simulink model "Kinematic_control"  (R2022b)
settings: Solver=FixedStepAuto  StartTime=0.0  StopTime=T_final  FixedStep=Ts  RelTol=1e-3
values from neighbouring files (symbols this model uses):
  BDD_thresh = 1    [Run_model.m]
  d = 0.1    [Run_model.m]
  I_single = sort(randperm(n_meas,n_attack)).'    [Run_model.m]
  kx = 15    [Run_model.m]
  ky = 15    [Run_model.m]
  max_iter = 2000    [Run_model.m]
  n_meas = 6    [Run_model.m]
  P_inp = 1e-10    [Run_model.m]
  R_meas = 1e-4    (= 0.0001)    [Run_model.m]
  Ts = 0.01    [Run_model.m]    (also in imu.m)
  u0 = zeros(n_int,1)    [Run_model.m]
  y0 = zeros(n_meas,1)    [Run_model.m]
  z_hat0 = z_initial    [Run_model.m]
  z_initial = [theta0;x0;y0]    [Run_model.m]
libraries: simulink x2, sharedTrackingLibrary x1
settings Model: Creator=Abelb  LastModifiedBy=Abelb

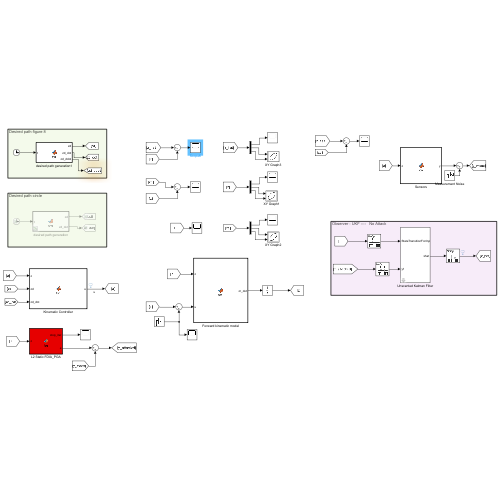
[thumbnail: Simulink's stored preview of the top-level diagram]
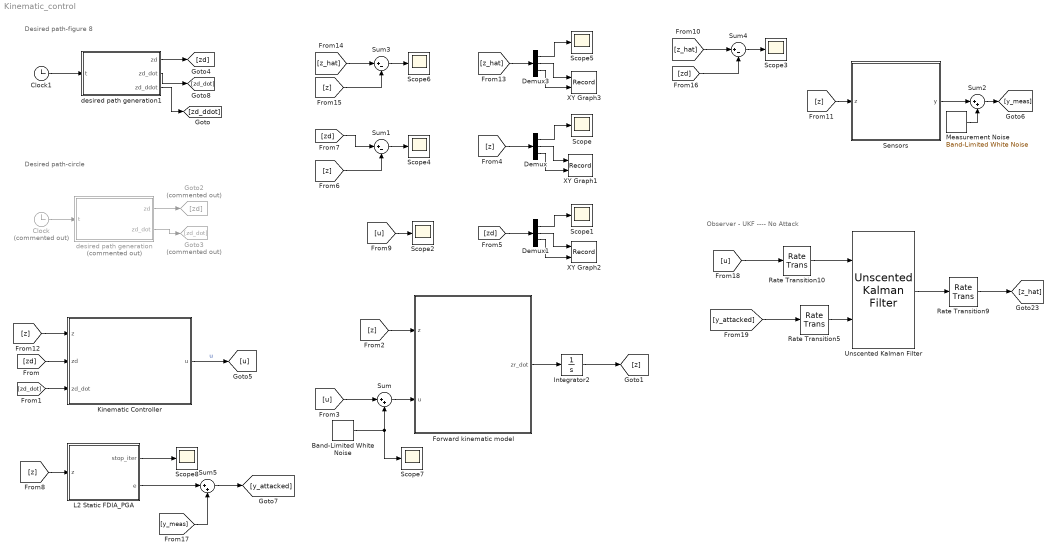
== system Kinematic_control ==
  note: Desired path-circle
  note: Desired path-figure 8
  note: Observer - UKF ---- No Attack
  Band-Limited White Noise : simulink/Sources/Band-Limited White Noise  Cov=P_inp*Ts  Ts=Ts  seed=[23341]
  Clock : Clock  Commented=on
  Clock1 : Clock
  Demux : Demux  Outputs=3
  Demux1 : Demux  Outputs=3
  Demux3 : Demux  Outputs=3
  Forward kinematic model : MATLAB Function  TreatAsAtomicUnit=on
  Goto2 : Goto  Commented=on  GotoTag=zd
  Goto3 : Goto  Commented=on  GotoTag=zd_dot
  Integrator2 : Integrator  InitialCondition=z_initial
  Kinematic Controller : MATLAB Function  TreatAsAtomicUnit=on
  L2 Static FDIA_PGA : MATLAB Function  TreatAsAtomicUnit=on
  Measurement Noise : simulink/Sources/Band-Limited White Noise  Cov=R_meas*Ts  Ts=Ts  seed=[23341]
  Rate Transition10 : RateTransition  InitialCondition=u0  OutPortSampleTime=Ts
  Rate Transition5 : RateTransition  InitialCondition=y0  OutPortSampleTime=Ts
  Rate Transition9 : RateTransition  InitialCondition=z_hat0  OutPortSampleTime=0
  Scope{,1..8} (9 alike) : Scope
  Sensors : MATLAB Function  TreatAsAtomicUnit=on
  Sum : Sum  Inputs=|++
  Sum1 : Sum  Inputs=|+-
  Sum2 : Sum  Inputs=|++
  Sum3 : Sum  Inputs=|+-
  Sum4 : Sum  Inputs=|+-
  Sum5 : Sum  Inputs=|++
  Unscented Kalman Filter : sharedTrackingLibrary/Unscented Kalman Filter  StateTransitionFcn=Dynamicfcn  HasAdditiveProcessNoise=Additive  ProcessNoise=P_diag  HasTimeVaryingProcessNoise=off  HasStateTransitionFcnExtraArgument=1  InitialState=z_hat0  InitialStateCovariance=1  Alpha=1e-3  Beta=2  Kappa=0  MeasurementFcn1=measurement_model  HasMeasurementEnablePort1=off  HasAdditiveMeasurementNoise1=Additive  MeasurementNoise1=R_diag  HasTimeVaryingMeasurementNoise1=off  HasMeasurementFcnExtraArgument1=0  HasMeasurementWrapping1=off  MeasurementFcn2=myMeasurementFcn  HasMeasurementEnablePort2=off  HasAdditiveMeasurementNoise2=Additive  MeasurementNoise2=1  HasTimeVaryingMeasurementNoise2=off  HasMeasurementFcnExtraArgument2=0  HasMeasurementWrapping2=off  MeasurementFcn3=myMeasurementFcn  HasMeasurementEnablePort3=off  HasAdditiveMeasurementNoise3=Additive  MeasurementNoise3=1  HasTimeVaryingMeasurementNoise3=off  HasMeasurementFcnExtraArgument3=0  HasMeasurementWrapping3=off  MeasurementFcn4=myMeasurementFcn  HasMeasurementEnablePort4=off  HasAdditiveMeasurementNoise4=Additive  MeasurementNoise4=1  HasTimeVaryingMeasurementNoise4=off  HasMeasurementFcnExtraArgument4=0  HasMeasurementWrapping4=off  MeasurementFcn5=myMeasurementFcn  HasMeasurementEnablePort5=off  HasAdditiveMeasurementNoise5=Additive  MeasurementNoise5=1  HasTimeVaryingMeasurementNoise5=off  HasMeasurementFcnExtraArgument5=0  HasMeasurementWrapping5=off  EnableMultirate=off  StateTransitionFcnSampleTime=1  MeasurementFcn1SampleTime=1  MeasurementFcn2SampleTime=1  MeasurementFcn3SampleTime=1  MeasurementFcn4SampleTime=1  MeasurementFcn5SampleTime=1  UseCurrentEstimator=on  OutputStateCovariance=off  DataType=double  SampleTime=Ts  NumberOfMeasurements=1
      settings: LibrarySourceBlock=cstblocks/State Estimation/Unscented Kalman Filter
  XY Graph1 : Record  FileSettingsInternal="{\"entries\":[{\"content\":{\"excelSettings\":{\"content\":{},\"type\":\"Streamout.ExcelSettings\"}},\"type\":\"Streamout.FileSettingStorage\",\"uuid\":\"01bd68c0-a6de-48cf-b19e-281f727054bd\"}],\"packageUris\":[\"http://schema.mathworks.com/mf0/streamout_blocks/R2020a\"],\"version\":\"1.0\"}"  Layout=[1 1]  SignalsInternal="{\"entries\":[{\"content\":{\"signals\":[{\"content\":{\"blockPath\":[\"Kinematic_control/XY Graph1\"],\"channel\":[],\"dimensions\":[1],\"domain\":\"Kinematic_control/XY Graph1\",\"lineColor\":\"#a2142f\",\"plots\":[1],\"port\":1,\"sid\":[\"\"],\"signalID\":27670,\"signalName\":\"Demux:2\"},\"type\":\"RecordBlkView.Signal\",\"uuid\":\"26d08ffc-2588-4001-8cc0-8bd54fef36d5\"},{\"content\":{\"blockPath\":[\"Kinematic_control/XY Graph1\"],\"channel\":[],\"dimensions\":[1],\"domain\":\"Kinematic_control/XY Graph1\",\"lineColor\":\"#139fff\",\"plots\":[1],\"port\":2,\"sid\":[\"\"],\"signalID\":27674,\"signalName\":\"Demux:3\"},\"type\":\"RecordBlkView.Signal\",\"uuid\":\"b11bfe9c-7795-424d-906e-92d6e4f2295a\"}]},\"type\":\"RecordBlkView.InputSignals\",\"uuid\":\"246071f6-524c-4d09-8024-359ba633c286\"}],\"packageUris\":[\"http://schema.mathworks.com/mf0/streamout_blocks/R2020a\"],\"version\":\"1.0\"}"  VisualizationBindings="{\"xyplotplugin\":{\"info\":[{\"series\":[{\"bindingParametersList\":[{\"parameter\":\"X-Axis\",\"signalID\":27670,\"signalName\":\"Demux:2\"},{\"parameter\":\"Y-Axis\",\"signalID\":27674,\"signalName\":\"Demux:3\"}],\"seriesID\":37825}],\"subplotID\":1}]}}"  CompatibilityTag=XY
  XY Graph2 : Record  FileSettingsInternal="{\"entries\":[{\"content\":{\"excelSettings\":{\"content\":{},\"type\":\"Streamout.ExcelSettings\"}},\"type\":\"Streamout.FileSettingStorage\",\"uuid\":\"0abfc6d3-6f78-40e7-b734-c86787280a0b\"}],\"packageUris\":[\"http://schema.mathworks.com/mf0/streamout_blocks/R2020a\"],\"version\":\"1.0\"}"  Layout=[1 1]  SignalsInternal="{\"entries\":[{\"content\":{\"signals\":[{\"content\":{\"blockPath\":[\"Kinematic_control/XY Graph2\"],\"channel\":[],\"dimensions\":[1],\"domain\":\"Kinematic_control/XY Graph2\",\"lineColor\":\"#a2142f\",\"plots\":[1],\"port\":1,\"sid\":[\"\"],\"signalID\":27678,\"signalName\":\"Demux1:2\"},\"type\":\"RecordBlkView.Signal\",\"uuid\":\"806e5a49-1a7f-4b20-bf57-f9789684ac96\"},{\"content\":{\"blockPath\":[\"Kinematic_control/XY Graph2\"],\"channel\":[],\"dimensions\":[1],\"domain\":\"Kinematic_control/XY Graph2\",\"lineColor\":\"#139fff\",\"plots\":[1],\"port\":2,\"sid\":[\"\"],\"signalID\":27682,\"signalName\":\"Demux1:3\"},\"type\":\"RecordBlkView.Signal\",\"uuid\":\"c86d3bda-4c51-4fac-93a7-c805a71bfe79\"}]},\"type\":\"RecordBlkView.InputSignals\",\"uuid\":\"8dc29a48-8473-4681-ba67-f4f4004b7990\"}],\"packageUris\":[\"http://schema.mathworks.com/mf0/streamout_blocks/R2020a\"],\"version\":\"1.0\"}"  VisualizationBindings="{\"xyplotplugin\":{\"info\":[{\"series\":[{\"bindingParametersList\":[{\"parameter\":\"X-Axis\",\"signalID\":27678,\"signalName\":\"Demux1:2\"},{\"parameter\":\"Y-Axis\",\"signalID\":27682,\"signalName\":\"Demux1:3\"}],\"seriesID\":29925}],\"subplotID\":1}]}}"  CompatibilityTag=XY
  XY Graph3 : Record  FileSettingsInternal="{\"entries\":[{\"content\":{\"excelSettings\":{\"content\":{},\"type\":\"Streamout.ExcelSettings\"}},\"type\":\"Streamout.FileSettingStorage\",\"uuid\":\"af403117-8c54-4f65-b15d-aaba59cdf658\"}],\"packageUris\":[\"http://schema.mathworks.com/mf0/streamout_blocks/R2020a\"],\"version\":\"1.0\"}"  Layout=[1 1]  SignalsInternal="{\"entries\":[{\"content\":{\"signals\":[{\"content\":{\"blockPath\":[\"Kinematic_control/XY Graph3\"],\"channel\":[],\"dimensions\":[1],\"domain\":\"Kinematic_control/XY Graph3\",\"lineColor\":\"#a2142f\",\"plots\":[1],\"port\":1,\"sid\":[\"\"],\"signalID\":27686,\"signalName\":\"Demux3:2\"},\"type\":\"RecordBlkView.Signal\",\"uuid\":\"5509430a-c9ff-4fe5-b9f4-7d88396fb61c\"},{\"content\":{\"blockPath\":[\"Kinematic_control/XY Graph3\"],\"channel\":[],\"dimensions\":[1],\"domain\":\"Kinematic_control/XY Graph3\",\"lineColor\":\"#139fff\",\"plots\":[1],\"port\":2,\"sid\":[\"\"],\"signalID\":27690,\"signalName\":\"Demux3:3\"},\"type\":\"RecordBlkView.Signal\",\"uuid\":\"e1d6a1c6-67ff-46a7-ad56-22e1f4e40b56\"}]},\"type\":\"RecordBlkView.InputSignals\",\"uuid\":\"e44e6304-3954-466c-be07-2fe59975f87a\"}],\"packageUris\":[\"http://schema.mathworks.com/mf0/streamout_blocks/R2020a\"],\"version\":\"1.0\"}"  VisualizationBindings="{\"xyplotplugin\":{\"info\":[{\"series\":[{\"bindingParametersList\":[{\"parameter\":\"X-Axis\",\"signalID\":27686,\"signalName\":\"Demux3:2\"},{\"parameter\":\"Y-Axis\",\"signalID\":27690,\"signalName\":\"Demux3:3\"}],\"seriesID\":53395}],\"subplotID\":1}]}}"  CompatibilityTag=XY
  desired path generation : MATLAB Function  Commented=on  TreatAsAtomicUnit=on
  desired path generation1 : MATLAB Function  TreatAsAtomicUnit=on
  wires:
  Forward kinematic model/1(zr_dot) -> Integrator2/1
  desired path generation1/3(zd_ddot) -> [zd_ddot]
  Clock1/1 -> desired path generation1/1(t)
  desired path generation1/2(zd_dot) -> [zd_dot]
  desired path generation1/1(zd) -> [zd]
  desired path generation/2(zd_dot) -> Goto3/1
  desired path generation/1(zd) -> Goto2/1
  Clock/1 -> desired path generation/1(t)
  [zd] -> Kinematic Controller/2(zd)
  [zd_dot] -> Kinematic Controller/3(zd_dot)
  Integrator2/1 -> [z]
  [z] -> Forward kinematic model/1(z)
  [z] -> Demux/1
  Demux/1 -> Scope/1
  Demux/2 -> XY Graph1/1
  Demux/3 -> XY Graph1/2
  Demux1/2 -> XY Graph2/1
  Demux1/3 -> XY Graph2/2
  [zd] -> Demux1/1
  Demux1/1 -> Scope1/1
  Kinematic Controller/1(u) -> [u]  "u"
  [zd] -> Sum1/1
  [z] -> Sum1/2
  Sum1/1 -> Scope4/1
  Unscented Kalman Filter/1 -> Rate Transition9/1
  Rate Transition9/1 -> [z_hat]
  Rate Transition10/1 -> Unscented Kalman Filter/1
  Rate Transition5/1 -> Unscented Kalman Filter/2
  [u] -> Rate Transition10/1
  [u] -> Scope2/1
  [z] -> Sensors/1(z)
  Measurement Noise/1 -> Sum2/2
  Demux3/2 -> XY Graph3/1
  Demux3/1 -> Scope5/1
  Demux3/3 -> XY Graph3/2
  [z_hat] -> Demux3/1
  [z] -> Sum3/2
  [z_hat] -> Sum3/1
  Sum3/1 -> Scope6/1
  [y_attacked] -> Rate Transition5/1
  Sensors/1(y) -> Sum2/1
  Sum2/1 -> [y_meas]
  Sum4/1 -> Scope3/1
  [zd] -> Sum4/2
  [z_hat] -> Sum4/1
  [z] -> Kinematic Controller/1(z)
  Sum/1 -> Forward kinematic model/2(u)
  [u] -> Sum/1
  Band-Limited White Noise/1 -> Scope7/1, Sum/2
  L2 Static FDIA_PGA/2(e) -> Sum5/1
  L2 Static FDIA_PGA/1(stop_iter) -> Scope8/1
  [y_meas] -> Sum5/2
  Sum5/1 -> [y_attacked]
  [z] -> L2 Static FDIA_PGA/1(z)

== matlab function Kinematic_control/desired path generation1 ==
  data: t input; zd output; zd_dot output; zd_ddot output
function [zd,zd_dot,zd_ddot] = fcn(t)

t = t/10;

a=1;
x = a*cos(t)/(1+sin(t)^2);
y = a*sin(t)*cos(t)/(1+sin(t)^2);
% unit circle (radius = 1; origin: (0,0))
zd = [atan(y./x);              % theta
      a*cos(t)/(1+sin(t)^2);         % x
      a*sin(t)*cos(t)/(1+sin(t)^2)];        % y

zd_dot = [ 0;
          -a*sin(t)*(cos(t)^2+2)/(1+sin(t)^2)^2;
          (a*cos(t)^2-2*a*sin(t)^2)/(1+sin(t)^2)^2];

z1 = (a*sin(t)^2*cos(t)^3-11*a*cos(t)^3+8*a*cos(t))/(1+sin(t)^2)^3;
z2 = -2*a*sin(t)*cos(t)*(3+2*cos(t)^2-sin(t)^2)/(1+sin(t)^2)^3;
zd_ddot = [z1;
           z2];

== matlab function Kinematic_control/Kinematic Controller ==
  data: z input; u output; zd input; zd_dot input; d parameter; kx parameter; ky parameter
function u = fcn(z,zd,zd_dot,d, kx, ky)

%% unpacking inputs
theta = z(1);
x = z(2);
y = z(3);
xd = zd(2);
yd = zd(3);
xd_dot = zd_dot(2);
yd_dot = zd_dot(3);



%% controller
K1 = [cos(theta) sin(theta);
     -sin(theta)/d cos(theta)/d];
K2 = [xd_dot + kx*(xd-x) ;
      yd_dot + ky*(yd-y)];
u = K1*K2;



%% rate constraint (physics)
v = u(1);
omega = u(2);

%% packing output
u = [v;
     omega];

== matlab function Kinematic_control/Sensors ==
  data: z input; y output; n_meas parameter
function y = fcn(z,n_meas)

coder.extrinsic('measurement_model');

y = zeros(n_meas,1);
y(:) = measurement_model(z);

== matlab function Kinematic_control/Forward kinematic model ==
  data: z input; u input; zr_dot output; d parameter
function zr_dot = fcn(z,u,d)

%% unpacking the state vectors
theta=z(1);

%% unpacking the intput
v=u(1);
omega=u(2);

%% ODE
theta_dot=omega;
x_dot=v*cos(theta)-d*omega*sin(theta);
y_dot=v*sin(theta)+d*omega*cos(theta);
% phir_dot = (v+omega)/r;
% phil_dot = (v-omega)/r;


%% packing the output
zr_dot=[theta_dot;x_dot;y_dot];

== matlab function Kinematic_control/L2 Static FDIA_PGA ==
  data: stop_iter output; I_single parameter; e output; BDD_thresh parameter; max_iter parameter; z input; n_meas parameter
function [stop_iter,e]  = fcn(I_single,BDD_thresh,max_iter, z,n_meas)

coder.extrinsic('L2_FDIA2');
%% Measurement Channel Attack
%  Assumptions:
%  1. The attacker knows the actual measurement
%  2. The attacker can only corrupt upto n_attack measurements
%  3. The attacker knows the BDD theshold

attack_idx = I_single;
% e = L2_FDIA(C_obsv_d,attack_idx,0.9*BDD_thresh);

L=0.235/2;  %1/2 distance between two wheels,(m)
r=0.05;     %radius of wheels,(m)

C = @(x,y,theta) [-x*sin(theta) cos(theta) 0;
                   y*cos(theta) 0 sin(theta);
                   0 1 0;
                   0 0 1;
                   0 1/(4*r) L/(4*r);
                   0 1/(4*r) -L/(4*r)];
Cd = C(z(2),z(3),z(1));

e = zeros(n_meas,1);
stop_iter = 0;
[stop_iter(:),e(:)] = L2_FDIA2(Cd,attack_idx,BDD_thresh,max_iter);

== matlab function Kinematic_control/desired path generation ==
  data: t input; zd output; zd_dot output
function [zd,zd_dot] = fcn(t)

 t = t/10;


% unit circle (radius = 1; origin: (0,0))
zd = [t;
      sin(t);         % x
      -1*cos(t)];        % y

zd_dot = [1;
          1*cos(t) ;
          1*sin(t) ];
